simulink model "MDCC"  (R2021b)
settings: Solver=FixedStepDiscrete  StartTime=0.0  StopTime=10.0  FixedStep=0.0001  RelTol=1e-3
model workspace (MATLAB code in the model file):
  | cmdLim = Simulink.Parameter;
  | cmdLim.Value = 15;
  | cmdLim.Description = 'Limit for controlling the maximum surface command angle.';
  | cmdLim.Min = 0;
  | cmdLim.Max = 90;
  | cmdLim.DocUnits = 'deg';
  | 
  | dispGain = Simulink.Parameter;
  | dispGain.Value = 0.75;
  | dispGain.Description = 'Gain applied to the displacement error.';
  | dispGain.Min = 0;
  | dispGain.Max = [];
  | dispGain.DocUnits = 'deg/sec/deg';
  | 
  | dispLim = Simulink.Parameter;
  | dispLim.Value = 30;
  | dispLim.Description = 'Limit for controlling the maximum commanded angle.';
  | dispLim.Min = 0;
  | dispLim.Max = 180;
  | dispLim.DocUnits = 'deg';
  | 
  | intGain = Simulink.Parameter;
  | intGain.Value = 0.5;
  | intGain.Description = 'Gain applied to the integral error.';
  | intGain.Min = 0;
  | intGain.Max = [];
  | intGain.DocUnits = 'deg/sec/deg/sec';
  | 
  | intLim = Simulink.Parameter;
  | intLim.Value = 5;
  | intLim.Description = 'Limit for controlling the maximum commanded angle.';
  | intLim.Min = 0;
  | intLim.Max = 90;
  | intLim.DocUnits = 'deg';
  | 
  | rateGain = Simulink.Parameter;
  | rateGain.Value = 2;
  | rateGain.Description = 'Gain applied to the rate error.';
  | rateGain.Min = 0;
  | rateGain.Max = [];
  | rateGain.DocUnits = 'deg/deg/sec';
  | 
  | rateLim = Simulink.Parameter;
  | rateLim.Value = 6;
  | rateLim.Description = 'Limit for controlling the maximum commanded angle.';
  | rateLim.Min = 0;
  | rateLim.Max = 180;
  | rateLim.DocUnits = 'deg/sec';
  | 
  | hdgGain = Simulink.Parameter;
  | hdgGain.Value = 0.015;
values from neighbouring files (symbols this model uses):
  KfDeadCompen_SetDeltaTime_us = myPackage.Parameter    [DeadCompen.m]
  Ts = 5E-6    (= 5e-06)    [iPMSM_data.m]
  VbDeadComp_SwtUseIsttrDes_flg = myPackage.Parameter    [DeadCompen.m]
  VfDeadCompen_ISttrDdeThdSwt_A = myPackage.Parameter    [DeadCompen.m]
  VfDeadCompen_ISttrIgbtThdSwt_A = myPackage.Parameter    [DeadCompen.m]
  VfDeadCompen_rDdeISttrHi_R = myPackage.Parameter    [DeadCompen.m]
  VfDeadCompen_rDdeISttrLo_R = myPackage.Parameter    [DeadCompen.m]
  VfDeadCompen_rIgbtISttrHi_R = myPackage.Parameter    [DeadCompen.m]
  VfDeadCompen_rIgbtISttrLo_R = myPackage.Parameter    [DeadCompen.m]
  VfDeadCompen_uDdeISttrHi_V = myPackage.Parameter    [DeadCompen.m]
  VfDeadCompen_uDdeISttrLo_V = myPackage.Parameter    [DeadCompen.m]
  VfDeadCompen_uIgbtISttrHi_V = myPackage.Parameter    [DeadCompen.m]
  VfDeadCompen_uIgbtISttrLo_V = myPackage.Parameter    [DeadCompen.m]
undefined symbols (not defined in the file or in its folder): CosTable12bit_Y, GLBCal_GLBCal_Kf_DCLinkOverVolErrThd_V, GLBCal_GLBCal_Kf_DCLinkUnderVolErrThd_V, GLBCal_GLBCal_Kf_EquiLd_NULL, GLBCal_GLBCal_Kf_EquiLq_NULL, GLBCal_GLBCal_Kf_MotorRatedSpeed_rpm, GLBCal_GLBCal_Kf_MotorSpeedHysteresis_Coef, GLBCal_Ke_MotorPolePairsNum_NULL, IoHwAbOpArg_PwmDutyCyclePhU_NULL, IoHwAbOpArg_PwmDutyCyclePhV_NULL, IoHwAbOpArg_PwmDutyCyclePhW_NULL, IoHwAbOpArg_PwmOutputEn, KbMDCC_DeadTimeCompEn_flg, KbMDCC_MCF_flgHarmInIsdqTab11ZR_flg, KbMDCC_MCF_flgHarmInIsdqTab13ZR_flg, KbMDCC_MCF_flgHarmInIsdqTab5ZR_flg, KbMDCC_MCF_flgHarmInIsdqTab7ZR_flg, KbMDCC_MCF_flgHarmInject_flg, KbMDCC_SetEAngleEn_flg, KbMDCC_UdUqFwOmit_flg, KfDeadCompen_CpPeriodTimesT_NULL, KfMDCC_ActiveDischargeIdCurVal_A, KfMDCC_ActiveDischargeIqCurVal_A, KfMDCC_DCLinkVolRate_coef, KfMDCC_DebugEAngleInit_rad, KfMDCC_DebugUalphaVolCmd_V, KfMDCC_DebugUbetaVolCmd_V, KfMDCC_DebugUdCmd_V, KfMDCC_DebugUqCmd_V, KfMDCC_DebugUsCmd_V, KfMDCC_DebugUsRate_V, KfMDCC_IMCResp_NULL, KfMDCC_IMCStab_NULL, KfMDCC_InvParkCpPeriodTimesT_NULL, KfMDCC_MCF_CircAge_NULL, KfMDCC_MCF_flgUse11Harm_flg, KfMDCC_MCF_flgUse13Harm_flg, KfMDCC_MCF_flgUse5Harm_flg, KfMDCC_MCF_flgUse7Harm_flg, KfMDCC_MCF_Harm1113FLParamSpeedThrd_rads, KfMDCC_MCF_Harm57FLParamSpeedThrd_rads, KfMDCC_MCF_HarmcofFltN_NULL, KfMDCC_MCF_HarmCpnAg_NULL, KfMDCC_MCF_HarmfLParaHigh_coef, KfMDCC_MCF_HarmfLParaLow_coef, KfMDCC_MCF_HarmIn1113ZRY_Trq_Nm, KfMDCC_MCF_HarmIn11_SpdLimHigh_rads, KfMDCC_MCF_HarmIn11_SpdLimLow_rads, KfMDCC_MCF_HarmIn11ZRY_Isd_A, KfMDCC_MCF_HarmIn11ZRY_Isq_A, KfMDCC_MCF_HarmIn13_SpdLimHigh_rads, KfMDCC_MCF_HarmIn13_SpdLimLow_rads, KfMDCC_MCF_HarmIn13ZRY_Isd_A, KfMDCC_MCF_HarmIn13ZRY_Isq_A, KfMDCC_MCF_HarmIn57ZRY_Trq_Nm, KfMDCC_MCF_HarmIn5_SpdLimHigh_rads, KfMDCC_MCF_HarmIn5_SpdLimLow_rads, KfMDCC_MCF_HarmIn5ZRY_Isd_A, KfMDCC_MCF_HarmIn5ZRY_Isq_A, KfMDCC_MCF_HarmIn7_SpdLimHigh_rads ... (+47)
libraries: simulink x40, PMSM_Library x3, mcbcontrolslib x1
(part 7 of 8)

== system MDCC/DoCurCtr_sys/MDCC/UdUqCalc_Sys/MDCC_MCF_Sys/Enabled Subsystem/Subsystem1/Park5/Subsystem ==
  In1 : Inport
  MCF_dtPWM : Inport  Port=2
  dB_Harm : Inport  Port=3
  Add : Sum
  Add1 : Sum  Inputs=-+
  Add2 : Sum
  Constant1 : Constant  OutDataTypeStr=single
  Constant2 : Constant  Value=2*pi  OutDataTypeStr=single
  Constant4 : Constant  OutDataTypeStr=single
  Divide{,1..3} (4 alike) : Product  Inputs=**
  Divide4 : Product  Inputs=*/
  Unit Delay : UnitDelay  SampleTime=-1  HasFrameUpgradeWarning=on
  Out1 : Outport
  wires:
  Add/1 -> Out1/1, Unit Delay/1
  Divide/1 -> Add/1
  Constant1/1 -> Add1/2
  Add1/1 -> Divide1/1
  Constant2/1 -> Divide2/1
  MCF_dtPWM/1 -> Divide2/2
  dB_Harm/1 -> Divide3/1
  Divide2/1 -> Divide3/2
  Divide3/1 -> Add2/2
  Constant4/1 -> Add2/1, Divide4/1
  Add2/1 -> Divide4/2
  Divide4/1 -> Divide/2, Add1/1
  In1/1 -> Divide1/2
  Divide1/1 -> Add/2
  Unit Delay/1 -> Divide/1

== system MDCC/DoCurCtr_sys/MDCC/UdUqCalc_Sys/MDCC_MCF_Sys/Enabled Subsystem/Subsystem1/Park5/Subsystem1 ==
  dB_Harm : Inport
  MCF_dtPWM : Inport  Port=2
  In1 : Inport  Port=3
  Add : Sum
  Add1 : Sum  Inputs=-+
  Add2 : Sum
  Constant1 : Constant  OutDataTypeStr=single
  Constant2 : Constant  Value=2*pi  OutDataTypeStr=single
  Constant4 : Constant  OutDataTypeStr=single
  Divide{,1..3} (4 alike) : Product  Inputs=**
  Divide4 : Product  Inputs=*/
  Unit Delay : UnitDelay  SampleTime=-1  HasFrameUpgradeWarning=on
  Out1 : Outport
  wires:
  Unit Delay/1 -> Divide/1
  Divide1/1 -> Add/2
  In1/1 -> Divide1/2
  Divide4/1 -> Add1/1, Divide/2
  Add2/1 -> Divide4/2
  Constant4/1 -> Divide4/1, Add2/1
  Divide3/1 -> Add2/2
  Divide2/1 -> Divide3/2
  dB_Harm/1 -> Divide3/1
  MCF_dtPWM/1 -> Divide2/2
  Constant2/1 -> Divide2/1
  Add1/1 -> Divide1/1
  Constant1/1 -> Add1/2
  Divide/1 -> Add/1
  Add/1 -> Unit Delay/1, Out1/1

== system MDCC/DoCurCtr_sys/MDCC/UdUqCalc_Sys/MDCC_MCF_Sys/Enabled Subsystem/Subsystem1/Park7/Subsystem ==
  In1 : Inport
  MCF_dtPWM : Inport  Port=2
  dB_Harm : Inport  Port=3
  Add : Sum
  Add1 : Sum  Inputs=-+
  Add2 : Sum
  Constant1 : Constant  OutDataTypeStr=single
  Constant2 : Constant  Value=2*pi  OutDataTypeStr=single
  Constant4 : Constant  OutDataTypeStr=single
  Divide{,1..3} (4 alike) : Product  Inputs=**
  Divide4 : Product  Inputs=*/
  Unit Delay : UnitDelay  SampleTime=-1  HasFrameUpgradeWarning=on
  Out1 : Outport
  wires:
  Add/1 -> Out1/1, Unit Delay/1
  Divide/1 -> Add/1
  Constant1/1 -> Add1/2
  Add1/1 -> Divide1/1
  Constant2/1 -> Divide2/1
  MCF_dtPWM/1 -> Divide2/2
  dB_Harm/1 -> Divide3/1
  Divide2/1 -> Divide3/2
  Divide3/1 -> Add2/2
  Constant4/1 -> Add2/1, Divide4/1
  Add2/1 -> Divide4/2
  Divide4/1 -> Divide/2, Add1/1
  In1/1 -> Divide1/2
  Divide1/1 -> Add/2
  Unit Delay/1 -> Divide/1

== system MDCC/DoCurCtr_sys/MDCC/UdUqCalc_Sys/MDCC_MCF_Sys/Enabled Subsystem/Subsystem1/Park7/Subsystem1 ==
  dB_Harm : Inport
  MCF_dtPWM : Inport  Port=2
  In1 : Inport  Port=3
  Add : Sum
  Add1 : Sum  Inputs=-+
  Add2 : Sum
  Constant1 : Constant  OutDataTypeStr=single
  Constant2 : Constant  Value=2*pi  OutDataTypeStr=single
  Constant4 : Constant  OutDataTypeStr=single
  Divide{,1..3} (4 alike) : Product  Inputs=**
  Divide4 : Product  Inputs=*/
  Unit Delay : UnitDelay  SampleTime=-1  HasFrameUpgradeWarning=on
  Out1 : Outport
  wires:
  Unit Delay/1 -> Divide/1
  Divide1/1 -> Add/2
  In1/1 -> Divide1/2
  Divide4/1 -> Add1/1, Divide/2
  Add2/1 -> Divide4/2
  Constant4/1 -> Divide4/1, Add2/1
  Divide3/1 -> Add2/2
  Divide2/1 -> Divide3/2
  dB_Harm/1 -> Divide3/1
  MCF_dtPWM/1 -> Divide2/2
  Constant2/1 -> Divide2/1
  Add1/1 -> Divide1/1
  Constant1/1 -> Add1/2
  Divide/1 -> Add/1
  Add/1 -> Unit Delay/1, Out1/1

== system MDCC/DoCurCtr_sys/MDCC/UdUqCalc_Sys/MDCC_MCF_Sys/Enabled Subsystem/Subsystem1/Subsystem/LookUpEAngleCosSin1 ==
  VuMDCC_MotorPositionCnt_NULL : Inport  OutMin=[0]  OutMax=[4095]
  Constant2 : Constant  Value=CosTable12bit_Y
  Constant3 : Constant  Value=SinTable12bit_Y
  Direct Lookup Table (n-D) : LookupNDDirect  NumberOfTableDimensions=1  TableIsInput=on  Table=[4 5 6]  TableMax=[4096]
  Direct Lookup Table (n-D)1 : LookupNDDirect  NumberOfTableDimensions=1  TableIsInput=on  Table=[4 5 6]  TableMax=[4096]
  VfMDCC_EAngleCos_NULL : Outport
  VfMDCC_EAngleSin_NULL : Outport  Port=2
  wires:
  VuMDCC_MotorPositionCnt_NULL/1 -> Direct Lookup Table (n-D)/1, Direct Lookup Table (n-D)1/1
  Direct Lookup Table (n-D)/1 -> VfMDCC_EAngleCos_NULL/1
  Direct Lookup Table (n-D)1/1 -> VfMDCC_EAngleSin_NULL/1
  Constant2/1 -> Direct Lookup Table (n-D)/2
  Constant3/1 -> Direct Lookup Table (n-D)1/2

== system MDCC/DoCurCtr_sys/MDCC/UdUqCalc_Sys/MDCC_MCF_Sys/Enabled Subsystem/Subsystem1/Subsystem/LookUpEAngleCosSin2 ==
  VuMDCC_MotorPositionCnt_NULL : Inport  OutMin=[0]  OutMax=[4095]
  Constant2 : Constant  Value=CosTable12bit_Y
  Constant3 : Constant  Value=SinTable12bit_Y
  Direct Lookup Table (n-D) : LookupNDDirect  NumberOfTableDimensions=1  TableIsInput=on  Table=[4 5 6]  TableMax=[4096]
  Direct Lookup Table (n-D)1 : LookupNDDirect  NumberOfTableDimensions=1  TableIsInput=on  Table=[4 5 6]  TableMax=[4096]
  VfMDCC_EAngleCos_NULL : Outport
  VfMDCC_EAngleSin_NULL : Outport  Port=2
  wires:
  VuMDCC_MotorPositionCnt_NULL/1 -> Direct Lookup Table (n-D)/1, Direct Lookup Table (n-D)1/1
  Direct Lookup Table (n-D)/1 -> VfMDCC_EAngleCos_NULL/1
  Direct Lookup Table (n-D)1/1 -> VfMDCC_EAngleSin_NULL/1
  Constant2/1 -> Direct Lookup Table (n-D)/2
  Constant3/1 -> Direct Lookup Table (n-D)1/2

== system MDCC/DoCurCtr_sys/MDCC/UdUqCalc_Sys/MDCC_MCF_Sys/Enabled Subsystem/Subsystem1/Subsystem/LookUpEAngleCosSin3 ==
  VuMDCC_MotorPositionCnt_NULL : Inport  OutMin=[0]  OutMax=[4095]
  Constant2 : Constant  Value=CosTable12bit_Y
  Constant3 : Constant  Value=SinTable12bit_Y
  Direct Lookup Table (n-D) : LookupNDDirect  NumberOfTableDimensions=1  TableIsInput=on  Table=[4 5 6]  TableMax=[4096]
  Direct Lookup Table (n-D)1 : LookupNDDirect  NumberOfTableDimensions=1  TableIsInput=on  Table=[4 5 6]  TableMax=[4096]
  VfMDCC_EAngleCos_NULL : Outport
  VfMDCC_EAngleSin_NULL : Outport  Port=2
  wires:
  VuMDCC_MotorPositionCnt_NULL/1 -> Direct Lookup Table (n-D)/1, Direct Lookup Table (n-D)1/1
  Direct Lookup Table (n-D)/1 -> VfMDCC_EAngleCos_NULL/1
  Direct Lookup Table (n-D)1/1 -> VfMDCC_EAngleSin_NULL/1
  Constant2/1 -> Direct Lookup Table (n-D)/2
  Constant3/1 -> Direct Lookup Table (n-D)1/2

== system MDCC/DoCurCtr_sys/MDCC/UdUqCalc_Sys/MDCC_MCF_Sys/Enabled Subsystem/Subsystem1/Subsystem/LookUpEAngleCosSin5 ==
  VuMDCC_MotorPositionCnt_NULL : Inport  OutMin=[0]  OutMax=[4095]
  Constant2 : Constant  Value=CosTable12bit_Y
  Constant3 : Constant  Value=SinTable12bit_Y
  Direct Lookup Table (n-D) : LookupNDDirect  NumberOfTableDimensions=1  TableIsInput=on  Table=[4 5 6]  TableMax=[4096]
  Direct Lookup Table (n-D)1 : LookupNDDirect  NumberOfTableDimensions=1  TableIsInput=on  Table=[4 5 6]  TableMax=[4096]
  VfMDCC_EAngleCos_NULL : Outport
  VfMDCC_EAngleSin_NULL : Outport  Port=2
  wires:
  VuMDCC_MotorPositionCnt_NULL/1 -> Direct Lookup Table (n-D)/1, Direct Lookup Table (n-D)1/1
  Direct Lookup Table (n-D)/1 -> VfMDCC_EAngleCos_NULL/1
  Direct Lookup Table (n-D)1/1 -> VfMDCC_EAngleSin_NULL/1
  Constant2/1 -> Direct Lookup Table (n-D)/2
  Constant3/1 -> Direct Lookup Table (n-D)1/2

== system MDCC/DoCurCtr_sys/MDCC/UdUqCalc_Sys/MDCC_MCF_Sys/Enabled Subsystem/Subsystem2/Mcf_AgTranCalc11/LookUpEAngleCosSin2 ==
  VuMDCC_MotorPositionCnt_NULL : Inport  OutMin=[0]  OutMax=[4095]
  Constant2 : Constant  Value=CosTable12bit_Y
  Constant3 : Constant  Value=SinTable12bit_Y
  Direct Lookup Table (n-D) : LookupNDDirect  NumberOfTableDimensions=1  TableIsInput=on  Table=[4 5 6]  TableMax=[4096]
  Direct Lookup Table (n-D)1 : LookupNDDirect  NumberOfTableDimensions=1  TableIsInput=on  Table=[4 5 6]  TableMax=[4096]
  VfMDCC_EAngleCos_NULL : Outport
  VfMDCC_EAngleSin_NULL : Outport  Port=2
  wires:
  VuMDCC_MotorPositionCnt_NULL/1 -> Direct Lookup Table (n-D)/1, Direct Lookup Table (n-D)1/1
  Direct Lookup Table (n-D)/1 -> VfMDCC_EAngleCos_NULL/1
  Direct Lookup Table (n-D)1/1 -> VfMDCC_EAngleSin_NULL/1
  Constant2/1 -> Direct Lookup Table (n-D)/2
  Constant3/1 -> Direct Lookup Table (n-D)1/2

== system MDCC/DoCurCtr_sys/MDCC/UdUqCalc_Sys/MDCC_MCF_Sys/Enabled Subsystem/Subsystem2/Mcf_AgTranCalc13/LookUpEAngleCosSin2 ==
  VuMDCC_MotorPositionCnt_NULL : Inport  OutMin=[0]  OutMax=[4095]
  Constant2 : Constant  Value=CosTable12bit_Y
  Constant3 : Constant  Value=SinTable12bit_Y
  Direct Lookup Table (n-D) : LookupNDDirect  NumberOfTableDimensions=1  TableIsInput=on  Table=[4 5 6]  TableMax=[4096]
  Direct Lookup Table (n-D)1 : LookupNDDirect  NumberOfTableDimensions=1  TableIsInput=on  Table=[4 5 6]  TableMax=[4096]
  VfMDCC_EAngleCos_NULL : Outport
  VfMDCC_EAngleSin_NULL : Outport  Port=2
  wires:
  VuMDCC_MotorPositionCnt_NULL/1 -> Direct Lookup Table (n-D)/1, Direct Lookup Table (n-D)1/1
  Direct Lookup Table (n-D)/1 -> VfMDCC_EAngleCos_NULL/1
  Direct Lookup Table (n-D)1/1 -> VfMDCC_EAngleSin_NULL/1
  Constant2/1 -> Direct Lookup Table (n-D)/2
  Constant3/1 -> Direct Lookup Table (n-D)1/2

== system MDCC/DoCurCtr_sys/MDCC/UdUqCalc_Sys/MDCC_MCF_Sys/Enabled Subsystem/Subsystem2/Mcf_AgTranCalc5/LookUpEAngleCosSin2 ==
  VuMDCC_MotorPositionCnt_NULL : Inport  OutMin=[0]  OutMax=[4095]
  Constant2 : Constant  Value=CosTable12bit_Y
  Constant3 : Constant  Value=SinTable12bit_Y
  Direct Lookup Table (n-D) : LookupNDDirect  NumberOfTableDimensions=1  TableIsInput=on  Table=[4 5 6]  TableMax=[4096]
  Direct Lookup Table (n-D)1 : LookupNDDirect  NumberOfTableDimensions=1  TableIsInput=on  Table=[4 5 6]  TableMax=[4096]
  VfMDCC_EAngleCos_NULL : Outport
  VfMDCC_EAngleSin_NULL : Outport  Port=2
  wires:
  VuMDCC_MotorPositionCnt_NULL/1 -> Direct Lookup Table (n-D)/1, Direct Lookup Table (n-D)1/1
  Direct Lookup Table (n-D)/1 -> VfMDCC_EAngleCos_NULL/1
  Direct Lookup Table (n-D)1/1 -> VfMDCC_EAngleSin_NULL/1
  Constant2/1 -> Direct Lookup Table (n-D)/2
  Constant3/1 -> Direct Lookup Table (n-D)1/2

== system MDCC/DoCurCtr_sys/MDCC/UdUqCalc_Sys/MDCC_MCF_Sys/Enabled Subsystem/Subsystem2/Mcf_AgTranCalc7/LookUpEAngleCosSin2 ==
  VuMDCC_MotorPositionCnt_NULL : Inport  OutMin=[0]  OutMax=[4095]
  Constant2 : Constant  Value=CosTable12bit_Y
  Constant3 : Constant  Value=SinTable12bit_Y
  Direct Lookup Table (n-D) : LookupNDDirect  NumberOfTableDimensions=1  TableIsInput=on  Table=[4 5 6]  TableMax=[4096]
  Direct Lookup Table (n-D)1 : LookupNDDirect  NumberOfTableDimensions=1  TableIsInput=on  Table=[4 5 6]  TableMax=[4096]
  VfMDCC_EAngleCos_NULL : Outport
  VfMDCC_EAngleSin_NULL : Outport  Port=2
  wires:
  VuMDCC_MotorPositionCnt_NULL/1 -> Direct Lookup Table (n-D)/1, Direct Lookup Table (n-D)1/1
  Direct Lookup Table (n-D)/1 -> VfMDCC_EAngleCos_NULL/1
  Direct Lookup Table (n-D)1/1 -> VfMDCC_EAngleSin_NULL/1
  Constant2/1 -> Direct Lookup Table (n-D)/2
  Constant3/1 -> Direct Lookup Table (n-D)1/2

== system MDCC/DoCurCtr_sys/MDCC/UdUqCalc_Sys/MDCC_MCF_Sys/Enabled Subsystem/Subsystem2/Subsystem/First_LowPass ==
  MCF_n : Inport
  Add : Sum  Inputs=-+
  Add1 : Sum
  CAL_MCF_HarmcofFltN_f32 : Constant  Value=KfMDCC_MCF_HarmcofFltN_NULL
  Constant : Constant  OutDataTypeStr=single
  Product : Product
  Product1 : Product
  Unit Delay : UnitDelay  SampleTime=-1  HasFrameUpgradeWarning=on
  MCF_nFlt : Outport
  wires:
  MCF_n/1 -> Product/1
  CAL_MCF_HarmcofFltN_f32/1 -> Product/2, Add/1
  Constant/1 -> Add/2
  Add/1 -> Product1/1
  Product1/1 -> Add1/2
  Product/1 -> Add1/1
  Add1/1 -> Unit Delay/1, MCF_nFlt/1
  Unit Delay/1 -> Product1/2

== system MDCC/DoCurCtr_sys/MDCC/SVM_Calc/DeadComp_Sys/DeadTime_Calc/Tavon_Calc/ia/uDdeCalc/If Action Subsystem ==
  iPhaseAbs : Inport
  Action Port : ActionPort  ActionPortLabel=if(u1 == 1)
  Add : Sum
  Constant : Constant  Value=VfDeadCompen_uDdeISttrLo_V
  Constant1 : Constant  Value=VfDeadCompen_rDdeISttrLo_R
  Product : Product
  UDde : Outport
  wires:
  Constant/1 -> Add/1
  Constant1/1 -> Product/1
  iPhaseAbs/1 -> Product/2
  Product/1 -> Add/2
  Add/1 -> UDde/1

== system MDCC/DoCurCtr_sys/MDCC/SVM_Calc/DeadComp_Sys/DeadTime_Calc/Tavon_Calc/ia/uDdeCalc/If Action Subsystem1 ==
  iPhaseAbs : Inport
  Action Port : ActionPort  ActionPortLabel=else
  Add : Sum
  Constant : Constant  Value=VfDeadCompen_uDdeISttrHi_V
  Constant1 : Constant  Value=VfDeadCompen_rDdeISttrHi_R
  Product : Product
  UDde : Outport
  wires:
  iPhaseAbs/1 -> Product/2
  Constant/1 -> Add/1
  Add/1 -> UDde/1
  Constant1/1 -> Product/1
  Product/1 -> Add/2

== system MDCC/DoCurCtr_sys/MDCC/SVM_Calc/DeadComp_Sys/DeadTime_Calc/Tavon_Calc/ia/uIgbtCalc/If Action Subsystem ==
  iPhaseAbs : Inport
  Action Port : ActionPort  ActionPortLabel=if(u1 == 0)
  Add : Sum
  Constant : Constant  Value=VfDeadCompen_uIgbtISttrLo_V
  Constant1 : Constant  Value=VfDeadCompen_rIgbtISttrLo_R
  Product : Product
  uIgbt : Outport
  wires:
  Constant/1 -> Add/1
  Constant1/1 -> Product/1
  iPhaseAbs/1 -> Product/2
  Product/1 -> Add/2
  Add/1 -> uIgbt/1

== system MDCC/DoCurCtr_sys/MDCC/SVM_Calc/DeadComp_Sys/DeadTime_Calc/Tavon_Calc/ia/uIgbtCalc/If Action Subsystem1 ==
  iPhaseAbs : Inport
  Action Port : ActionPort  ActionPortLabel=else
  Add : Sum
  Constant : Constant  Value=VfDeadCompen_uIgbtISttrHi_V
  Constant1 : Constant  Value=VfDeadCompen_rIgbtISttrHi_R
  Product : Product
  uIgbt : Outport
  wires:
  iPhaseAbs/1 -> Product/2
  Constant/1 -> Add/1
  Add/1 -> uIgbt/1
  Constant1/1 -> Product/1
  Product/1 -> Add/2

== system MDCC/DoCurCtr_sys/MDCC/SVM_Calc/DeadComp_Sys/DeadTime_Calc/Tavon_Calc/ib/uDdeCalc/If Action Subsystem ==
  iPhaseAbs : Inport
  Action Port : ActionPort  ActionPortLabel=if(u1 == 1)
  Add : Sum
  Constant : Constant  Value=VfDeadCompen_uDdeISttrLo_V
  Constant1 : Constant  Value=VfDeadCompen_rDdeISttrLo_R
  Product : Product
  UDde : Outport
  wires:
  Constant/1 -> Add/1
  Constant1/1 -> Product/1
  iPhaseAbs/1 -> Product/2
  Product/1 -> Add/2
  Add/1 -> UDde/1

== system MDCC/DoCurCtr_sys/MDCC/SVM_Calc/DeadComp_Sys/DeadTime_Calc/Tavon_Calc/ib/uDdeCalc/If Action Subsystem1 ==
  iPhaseAbs : Inport
  Action Port : ActionPort  ActionPortLabel=else
  Add : Sum
  Constant : Constant  Value=VfDeadCompen_uDdeISttrHi_V
  Constant1 : Constant  Value=VfDeadCompen_rDdeISttrHi_R
  Product : Product
  UDde : Outport
  wires:
  iPhaseAbs/1 -> Product/2
  Constant/1 -> Add/1
  Add/1 -> UDde/1
  Constant1/1 -> Product/1
  Product/1 -> Add/2

== system MDCC/DoCurCtr_sys/MDCC/SVM_Calc/DeadComp_Sys/DeadTime_Calc/Tavon_Calc/ib/uIgbtCalc/If Action Subsystem ==
  iPhaseAbs : Inport
  Action Port : ActionPort  ActionPortLabel=if(u1 == 0)
  Add : Sum
  Constant : Constant  Value=VfDeadCompen_uIgbtISttrLo_V
  Constant1 : Constant  Value=VfDeadCompen_rIgbtISttrLo_R
  Product : Product
  uIgbt : Outport
  wires:
  Constant/1 -> Add/1
  Constant1/1 -> Product/1
  iPhaseAbs/1 -> Product/2
  Product/1 -> Add/2
  Add/1 -> uIgbt/1

== system MDCC/DoCurCtr_sys/MDCC/SVM_Calc/DeadComp_Sys/DeadTime_Calc/Tavon_Calc/ib/uIgbtCalc/If Action Subsystem1 ==
  iPhaseAbs : Inport
  Action Port : ActionPort  ActionPortLabel=else
  Add : Sum
  Constant : Constant  Value=VfDeadCompen_uIgbtISttrHi_V
  Constant1 : Constant  Value=VfDeadCompen_rIgbtISttrHi_R
  Product : Product
  uIgbt : Outport
  wires:
  iPhaseAbs/1 -> Product/2
  Constant/1 -> Add/1
  Add/1 -> uIgbt/1
  Constant1/1 -> Product/1
  Product/1 -> Add/2

== system MDCC/DoCurCtr_sys/MDCC/SVM_Calc/DeadComp_Sys/DeadTime_Calc/Tavon_Calc/ic/uDdeCalc/If Action Subsystem ==
  iPhaseAbs : Inport
  Action Port : ActionPort  ActionPortLabel=if(u1 == 1)
  Add : Sum
  Constant : Constant  Value=VfDeadCompen_uDdeISttrLo_V
  Constant1 : Constant  Value=VfDeadCompen_rDdeISttrLo_R
  Product : Product
  UDde : Outport
  wires:
  Constant/1 -> Add/1
  Constant1/1 -> Product/1
  iPhaseAbs/1 -> Product/2
  Product/1 -> Add/2
  Add/1 -> UDde/1

== system MDCC/DoCurCtr_sys/MDCC/SVM_Calc/DeadComp_Sys/DeadTime_Calc/Tavon_Calc/ic/uDdeCalc/If Action Subsystem1 ==
  iPhaseAbs : Inport
  Action Port : ActionPort  ActionPortLabel=else
  Add : Sum
  Constant : Constant  Value=VfDeadCompen_uDdeISttrHi_V
  Constant1 : Constant  Value=VfDeadCompen_rDdeISttrHi_R
  Product : Product
  UDde : Outport
  wires:
  iPhaseAbs/1 -> Product/2
  Constant/1 -> Add/1
  Add/1 -> UDde/1
  Constant1/1 -> Product/1
  Product/1 -> Add/2

== system MDCC/DoCurCtr_sys/MDCC/SVM_Calc/DeadComp_Sys/DeadTime_Calc/Tavon_Calc/ic/uIgbtCalc/If Action Subsystem ==
  iPhaseAbs : Inport
  Action Port : ActionPort  ActionPortLabel=if(u1 == 0)
  Add : Sum
  Constant : Constant  Value=VfDeadCompen_uIgbtISttrLo_V
  Constant1 : Constant  Value=VfDeadCompen_rIgbtISttrLo_R
  Product : Product
  uIgbt : Outport
  wires:
  Constant/1 -> Add/1
  Constant1/1 -> Product/1
  iPhaseAbs/1 -> Product/2
  Product/1 -> Add/2
  Add/1 -> uIgbt/1

== system MDCC/DoCurCtr_sys/MDCC/SVM_Calc/DeadComp_Sys/DeadTime_Calc/Tavon_Calc/ic/uIgbtCalc/If Action Subsystem1 ==
  iPhaseAbs : Inport
  Action Port : ActionPort  ActionPortLabel=else
  Add : Sum
  Constant : Constant  Value=VfDeadCompen_uIgbtISttrHi_V
  Constant1 : Constant  Value=VfDeadCompen_rIgbtISttrHi_R
  Product : Product
  uIgbt : Outport
  wires:
  iPhaseAbs/1 -> Product/2
  Constant/1 -> Add/1
  Add/1 -> uIgbt/1
  Constant1/1 -> Product/1
  Product/1 -> Add/2

== system MDCC/DoCurCtr_sys/MDCC/SVM_Calc/MDSA/SVM_PU/T1_T2_Calc/Subsystem2/If Action Subsystem2/If Action Subsystem2 ==
  T4_m : Inport
  T6_m : Inport  Port=2
  delta : Inport  Port=3
  Action Port : ActionPort  ActionPortLabel=if(u1 ~= 0)
  Add : Sum
  Add1 : Sum  Inputs=-+
  Constant : Constant  OutDataTypeStr=single
  Constant1 : Constant  Value=0  OutDataTypeStr=single
  Demux : Demux  Outputs=2
  Mux : Mux  Inputs=2
  Mux1 : Mux  Inputs=2
  Relational Operator : RelationalOperator  Operator=<=  OutDataTypeStr=boolean  RndMeth=Simplest
  Switch : Switch  Criteria=u2 > Threshold
  T1 : Outport
  T2 : Outport  Port=2
  wires:
  T6_m/1 -> Add1/2, Relational Operator/1
  delta/1 -> Add/1, Add1/1, Relational Operator/2
  Relational Operator/1 -> Switch/2
  Constant/1 -> Mux/1
  Constant1/1 -> Mux/2
  Mux/1 -> Switch/1
  T4_m/1 -> Add/2
  Add/1 -> Mux1/1
  Add1/1 -> Mux1/2
  Mux1/1 -> Switch/3
  Switch/1 -> Demux/1
  Demux/1 -> T1/1
  Demux/2 -> T2/1

== system MDCC/DoCurCtr_sys/MDCC/SVM_Calc/MDSA/SVM_PU/T1_T2_Calc/Subsystem2/If Action Subsystem2/If Action Subsystem3 ==
  T4_m : Inport
  T6_m : Inport  Port=2
  delta : Inport  Port=3
  Action Port : ActionPort  ActionPortLabel=else
  Add : Sum
  Add1 : Sum  Inputs=-+
  Constant : Constant  OutDataTypeStr=single
  Constant1 : Constant  Value=0  OutDataTypeStr=single
  Demux : Demux  Outputs=2
  Mux : Mux  Inputs=2
  Mux1 : Mux  Inputs=2
  Relational Operator : RelationalOperator  Operator=<=  OutDataTypeStr=boolean  RndMeth=Simplest
  Switch : Switch  Criteria=u2 > Threshold
  T1 : Outport
  T2 : Outport  Port=2
  wires:
  Mux1/1 -> Switch/3
  delta/1 -> Add/1, Add1/1, Relational Operator/2
  Add1/1 -> Mux1/2
  Mux/1 -> Switch/1
  Relational Operator/1 -> Switch/2
  Switch/1 -> Demux/1
  Constant1/1 -> Mux/2
  Add/1 -> Mux1/1
  Constant/1 -> Mux/1
  T4_m/1 -> Add1/2, Relational Operator/1
  T6_m/1 -> Add/2
  Demux/2 -> T1/1
  Demux/1 -> T2/1

== system MDCC/DoCurCtr_sys/MDCC/SVM_Calc/MDSA/SVPWM/vIntp_PWMFOC_CalTriCompValue/CalTabc/Cal_T1T2/Sec1 ==
  Bus_XYZ_IN : Inport
  Action Port : ActionPort  ActionPortLabel=case [ 1 ]:
  Bus Creator1 : BusCreator  Inputs=2
  Bus Selector : BusSelector  OutputSignals=Z,Y
  Signal Conversion : SignalConversion  OverrideOpt=off
  Signal Conversion1 : SignalConversion  OverrideOpt=off
  Bus_T1T2 : Outport
  wires:
  Signal Conversion1/1 -> Bus Creator1/2
  Signal Conversion/1 -> Bus Creator1/1
  Bus Selector/2 -> Signal Conversion1/1  "<Y>"
  Bus Selector/1 -> Signal Conversion/1  "<Z>"
  Bus_XYZ_IN/1 -> Bus Selector/1
  Bus Creator1/1 -> Bus_T1T2/1

== system MDCC/DoCurCtr_sys/MDCC/SVM_Calc/MDSA/SVPWM/vIntp_PWMFOC_CalTriCompValue/CalTabc/Cal_T1T2/Sec2 ==
  Bus_XYZ_IN : Inport
  Action Port : ActionPort  ActionPortLabel=case [ 2 ]:
  -1 : Constant  Value=-1
  Bus Creator1 : BusCreator  Inputs=2
  Bus Selector : BusSelector  OutputSignals=Y,X
  Data Type Conversion1 : DataTypeConversion
  Product1 : Product
  Signal Conversion1 : SignalConversion  OverrideOpt=off
  Bus_T1T2 : Outport
  wires:
  Signal Conversion1/1 -> Bus Creator1/1
  Bus_XYZ_IN/1 -> Bus Selector/1
  Bus Selector/1 -> Signal Conversion1/1  "<Y>"
  Bus Selector/2 -> Product1/1  "<X>"
  Bus Creator1/1 -> Bus_T1T2/1
  Product1/1 -> Bus Creator1/2
  Data Type Conversion1/1 -> Product1/2
  -1/1 -> Data Type Conversion1/1

== system MDCC/DoCurCtr_sys/MDCC/SVM_Calc/MDSA/SVPWM/vIntp_PWMFOC_CalTriCompValue/CalTabc/Cal_T1T2/Sec3 ==
  Bus_XYZ_IN : Inport
  Action Port : ActionPort  ActionPortLabel=case [ 3 ]:
  -1 : Constant  Value=-1
  Bus Creator1 : BusCreator  Inputs=2
  Bus Selector : BusSelector  OutputSignals=Z,X
  Data Type Conversion1 : DataTypeConversion
  Product1 : Product
  Signal Conversion1 : SignalConversion  OverrideOpt=off
  Bus_T1T2 : Outport
  wires:
  Signal Conversion1/1 -> Bus Creator1/2
  Data Type Conversion1/1 -> Product1/1
  Bus_XYZ_IN/1 -> Bus Selector/1
  Bus Creator1/1 -> Bus_T1T2/1
  Product1/1 -> Bus Creator1/1
  Bus Selector/1 -> Product1/2  "<Z>"
  -1/1 -> Data Type Conversion1/1
  Bus Selector/2 -> Signal Conversion1/1  "<X>"

== system MDCC/DoCurCtr_sys/MDCC/SVM_Calc/MDSA/SVPWM/vIntp_PWMFOC_CalTriCompValue/CalTabc/Cal_T1T2/Sec4 ==
  Bus_XYZ_IN : Inport
  Action Port : ActionPort  ActionPortLabel=case [ 4 ]:
  -1 : Constant  Value=-1
  Bus Creator1 : BusCreator  Inputs=2
  Bus Selector : BusSelector  OutputSignals=X,Z
  Data Type Conversion2 : DataTypeConversion
  Product1 : Product
  Signal Conversion1 : SignalConversion  OverrideOpt=off
  Bus_T1T2 : Outport
  wires:
  Signal Conversion1/1 -> Bus Creator1/2
  Data Type Conversion2/1 -> Product1/1
  Bus_XYZ_IN/1 -> Bus Selector/1
  Bus Selector/2 -> Signal Conversion1/1  "<Z>"
  Bus Creator1/1 -> Bus_T1T2/1
  Product1/1 -> Bus Creator1/1
  Bus Selector/1 -> Product1/2  "<X>"
  -1/1 -> Data Type Conversion2/1

== system MDCC/DoCurCtr_sys/MDCC/SVM_Calc/MDSA/SVPWM/vIntp_PWMFOC_CalTriCompValue/CalTabc/Cal_T1T2/Sec5 ==
  Bus_XYZ_IN : Inport
  Action Port : ActionPort  ActionPortLabel=case [ 5 ]:
  -1 : Constant  Value=-1
  Bus Creator1 : BusCreator  Inputs=2
  Bus Selector : BusSelector  OutputSignals=X,Y
  Data Type Conversion1 : DataTypeConversion
  Product1 : Product
  Signal Conversion1 : SignalConversion  OverrideOpt=off
  Bus_T1T2 : Outport
  wires:
  Signal Conversion1/1 -> Bus Creator1/1
  Bus_XYZ_IN/1 -> Bus Selector/1
  Bus Creator1/1 -> Bus_T1T2/1
  Product1/1 -> Bus Creator1/2
  Data Type Conversion1/1 -> Product1/2
  -1/1 -> Data Type Conversion1/1
  Bus Selector/2 -> Product1/1  "<Y>"
  Bus Selector/1 -> Signal Conversion1/1  "<X>"

== system MDCC/DoCurCtr_sys/MDCC/SVM_Calc/MDSA/SVPWM/vIntp_PWMFOC_CalTriCompValue/CalTabc/Cal_T1T2/Sec6 ==
  Bus_XYZ_IN : Inport
  Action Port : ActionPort  ActionPortLabel=case [ 6 ]:
  -1 : Constant  Value=-1
  -1_1 : Constant  Value=-1
  Bus Creator1 : BusCreator  Inputs=2
  Bus Selector : BusSelector  OutputSignals=Y,Z
  Data Type Conversion2 : DataTypeConversion
  Data Type Conversion3 : DataTypeConversion
  Product2 : Product
  Product3 : Product
  Bus_T1T2 : Outport
  wires:
  Data Type Conversion3/1 -> Product3/1
  Bus_XYZ_IN/1 -> Bus Selector/1
  Bus Creator1/1 -> Bus_T1T2/1
  Product3/1 -> Bus Creator1/1
  Product2/1 -> Bus Creator1/2
  Data Type Conversion2/1 -> Product2/2
  -1_1/1 -> Data Type Conversion2/1
  -1/1 -> Data Type Conversion3/1
  Bus Selector/1 -> Product3/2  "<Y>"
  Bus Selector/2 -> Product2/1  "<Z>"

== system MDCC/DoCurCtr_sys/MDCC/SVM_Calc/MDSA/SVPWM/vIntp_PWMFOC_CalTriCompValue/CalTabc/Cal_TabcValue/CalTabcValue ==
  note: 占空比
  Bus_T1T2_Adjusted_IN : Inport
  Bus_Ts_Vdc : Inport  Port=2
  Add : Sum  Inputs=+--
  Add1 : Sum
  Add2 : Sum
  Bus Creator : BusCreator  Inputs=3
  Bus Selector : BusSelector  OutputSignals=signal1,signal2
  Bus Selector1 : BusSelector  OutputSignals=signal1
  Bus Selector2 : BusSelector  OutputSignals=signal2
  Bus Selector3 : BusSelector  OutputSignals=Ts
  Bus Selector4 : BusSelector  OutputSignals=Ts
  Bus_Ts_Vdc2 : InportShadow  Port=2
  Data Type Conversion1 : DataTypeConversion
  Divide : Product  Inputs=*/
  Divide1 : Product  Inputs=*/
  Divide2 : Product  Inputs=*/
  Gain : Gain  Gain=1/4
  Gain1 : Gain  Gain=0.5
  Gain2 : Gain  Gain=0.5
  Gain3 : Gain  Gain=2
  Gain4 : Gain  Gain=2
  Gain5 : Gain  Gain=2
  Subtract : Sum  Inputs=+-
  Subtract1 : Sum  Inputs=+-
  Subtract2 : Sum  Inputs=+-
  Bus_Tabc : Outport  Description=高电平计数值
  wires:
  Bus Creator/1 -> Bus_Tabc/1
  [Tbon] -> Add2/1
  Bus Selector2/1 -> Gain2/1  "<signal2>"
  [Taon] -> Add1/1
  Bus Selector1/1 -> Gain1/1  "<signal1>"
  Add/1 -> Gain/1
  Bus Selector/2 -> Add/3  "<signal2>"
  Bus Selector/1 -> Add/2  "<signal1>"
  Bus Selector3/1 -> Data Type Conversion1/1  "<Ts>"
  Bus_T1T2_Adjusted_IN/1 -> Bus Selector/1, Bus Selector1/1, Bus Selector2/1
  Data Type Conversion1/1 -> Add/1
  Gain/1 -> Gain3/1, [Taon]
  Gain1/1 -> Add1/2
  Gain2/1 -> Add2/2
  Add1/1 -> Gain4/1, [Tbon]
  Add2/1 -> Gain5/1
  Gain3/1 -> Subtract/2
  Gain4/1 -> Subtract1/2
  Gain5/1 -> Subtract2/2
  Bus Selector4/1 -> Subtract1/1, Divide2/2, Subtract2/1, Divide1/2, Divide/2, Subtract/1  "<Ts>"
  Subtract1/1 -> Divide1/1
  Subtract/1 -> Divide/1
  Subtract2/1 -> Divide2/1
  Divide1/1 -> Bus Creator/2
  Divide/1 -> Bus Creator/1
  Divide2/1 -> Bus Creator/3
  Bus_Ts_Vdc/1 -> Bus Selector3/1
  Bus_Ts_Vdc2/1 -> Bus Selector4/1

== system MDCC/DoCurCtr_sys/MDCC/SVM_Calc/MDSA/SVPWM/vIntp_PWMFOC_CalTriCompValue/CalTabc/Cal_TabcValue/ManageT1T2 ==
  Bus_T1T2_IN : Inport
  Bus_Ts_Vdc : Inport  Port=2
  Add : Sum
  Bus Creator : BusCreator  Inputs=2
  Bus Selector : BusSelector  OutputSignals=signal1,signal2
  Bus Selector1 : BusSelector  OutputSignals=signal1,signal2
  Bus Selector2 : BusSelector  OutputSignals=signal1,signal2
  Bus Selector3 : BusSelector  OutputSignals=Ts
  Constant1 : Constant
  Data Type Conversion : DataTypeConversion
  Data Type Conversion1 : DataTypeConversion
  Divide : Product  Inputs=*/
  Relational Operator : RelationalOperator  Operator=>  OutDataTypeStr=boolean  RndMeth=Nearest
  Signal Conversion : SignalConversion  OverrideOpt=off
  Signal Conversion1 : SignalConversion  OverrideOpt=off
  Subsystem : Subsystem
  Switch : Switch  Criteria=u2 ~= 0  OutDataTypeStr=single  ZeroCross=off
  Switch1 : Switch  Criteria=u2 ~= 0  OutDataTypeStr=single  ZeroCross=off
  Bus_T1T2_Adjusted : Outport
  wires:
  Relational Operator/1 -> Switch1/2, Switch/2
  Divide/1 -> Relational Operator/2
  Add/1 -> Relational Operator/1
  Data Type Conversion1/1 -> Divide/1
  Data Type Conversion/1 -> Divide/2
  Constant1/1 -> Data Type Conversion/1
  Bus Selector/2 -> Add/2  "<signal2>"
  Bus Selector/1 -> Add/1  "<signal1>"
  Bus_T1T2_IN/1 -> Signal Conversion/1, Bus Selector/1, Signal Conversion1/1
  Signal Conversion1/1 -> Subsystem/1(Bus_T1T2_IN)
  Signal Conversion/1 -> Bus Selector1/1
  Subsystem/1(Out1) -> Bus Selector2/1
  Bus Selector1/1 -> Switch/3  "<signal1>"
  Bus Selector2/1 -> Switch/1  "<signal1>"
  Switch/1 -> Bus Creator/1
  Bus Selector2/2 -> Switch1/1  "<signal2>"
  Bus Selector1/2 -> Switch1/3  "<signal2>"
  Switch1/1 -> Bus Creator/2
  Bus Creator/1 -> Bus_T1T2_Adjusted/1
  Bus_Ts_Vdc/1 -> [Bus_Ts_Vdc_ManageT1T2]
  [Bus_Ts_Vdc_ManageT1T2] -> Bus Selector3/1
  Bus Selector3/1 -> Data Type Conversion1/1  "<Ts>"
  [Bus_Ts_Vdc_ManageT1T2] -> Subsystem/2(Bus_Ts_Vdc)

== system MDCC/DoCurCtr_sys/MDCC/UdUqCalc_Sys/MDCC_MCF_Sys/Enabled Subsystem/Harmonic_Injection_11/Subsystem/Harm_11Step_KpKi/Harm11_KpKi_Table ==
  Rdc_absnWoFlt_rads : Inport
  1-D Lookup Table : Lookup_n-D  NumberOfTableDimensions=1  BreakpointsForDimension1=KfMDCC_MCF_Harmonic1113_KpKi_Spd_rads  Table=KfMDCC_MCF_Harmonic11_Kp_coef  InternalRulePriority=Speed  RndMeth=Simplest  InputSameDT=on
  1-D Lookup Table1 : Lookup_n-D  NumberOfTableDimensions=1  BreakpointsForDimension1=KfMDCC_MCF_Harmonic1113_KpKi_Spd_rads  Table=KfMDCC_MCF_Harmonic11_Ki_coef  InternalRulePriority=Speed  RndMeth=Simplest  InputSameDT=on
  Gain : Gain  Gain=0.11e-4
  MCF_Harm11_Kp : Outport  VectorParamsAs1DForOutWhenUnconnected=off
  MCF_Harm11_Ki : Outport  Port=2  VectorParamsAs1DForOutWhenUnconnected=off
  wires:
  1-D Lookup Table/1 -> MCF_Harm11_Kp/1
  1-D Lookup Table1/1 -> Gain/1
  Rdc_absnWoFlt_rads/1 -> 1-D Lookup Table1/1, 1-D Lookup Table/1
  Gain/1 -> MCF_Harm11_Ki/1

== system MDCC/DoCurCtr_sys/MDCC/UdUqCalc_Sys/MDCC_MCF_Sys/Enabled Subsystem/Harmonic_Injection_11/Subsystem/Harm_11Step_KpKi/Harm_11Step_daxis_PI ==
  MCF_Harm_isdDes11 : Inport
  MCF_Harm_isdAct11 : Inport  Port=2
  MCF_Harm_Kp : Inport  Port=3
  MCF_Harm_Ki : Inport  Port=4
  MCF_flgHarm11PIRest : Inport  Port=5
  Add : Sum  Inputs=+-
  Add1 : Sum  Inputs=+-
  Add2 : Sum  Inputs=+++
  Constant : Constant  Value=0  OutDataTypeStr=single
  Constant1 : Constant  Value=-KfMDCC_MCF_HarmonicInUDesMax_V
  Constant3 : Constant  Value=KfMDCC_MCF_HarmonicInUDesMax_V
  Product : Product
  Product1 : Product
  Saturation : simulink/Discontinuities/Saturation Dynamic  OutMin=[]  OutMax=[]  OutDataTypeStr=Inherit: Same as second input  OutDataType=fixdt(1, 16)  OutScaling=2^-10  DoSatur=off
      link override Data Type Propagation: ValuesUsedBestPrec=[11 -11]
  Switch : Switch  Criteria=u2 ~= 0
  Unit Delay : UnitDelay  SampleTime=-1  HasFrameUpgradeWarning=on
  Unit Delay1 : UnitDelay  SampleTime=-1  HasFrameUpgradeWarning=on
  MCF_Harm_ud11PI : Outport  VectorParamsAs1DForOutWhenUnconnected=off
  wires:
  MCF_Harm_isdAct11/1 -> Add/2
  MCF_Harm_isdDes11/1 -> Add/1
  MCF_Harm_Ki/1 -> Product1/2
  Switch/1 -> Add2/3
  Product/1 -> Add2/1
  Product1/1 -> Add2/2
  MCF_Harm_Kp/1 -> Product/2
  Add1/1 -> Product/1
  Unit Delay/1 -> Add1/2
  Add/1 -> Add1/1, Unit Delay/1, Product1/1
  Add2/1 -> Saturation/2
  Saturation/1 -> Unit Delay1/1, MCF_Harm_ud11PI/1
  Constant3/1 -> Saturation/1
  Constant1/1 -> Saturation/3
  MCF_flgHarm11PIRest/1 -> Switch/2
  Constant/1 -> Switch/3
  Unit Delay1/1 -> Switch/1

== system MDCC/DoCurCtr_sys/MDCC/UdUqCalc_Sys/MDCC_MCF_Sys/Enabled Subsystem/Harmonic_Injection_11/Subsystem/Harm_11Step_KpKi/Harm_11Step_qaxis_PI ==
  MCF_Harm_isqDes11 : Inport
  MCF_Harm_isqAct11 : Inport  Port=2
  MCF_Harm_Kp : Inport  Port=3
  MCF_Harm_Ki : Inport  Port=4
  MCF_flgHarm11PIRest : Inport  Port=5
  Add : Sum  Inputs=+-
  Add1 : Sum  Inputs=+-
  Add2 : Sum  Inputs=+++
  Constant : Constant  Value=0  OutDataTypeStr=single
  Constant1 : Constant  Value=-KfMDCC_MCF_HarmonicInUDesMax_V
  Constant3 : Constant  Value=KfMDCC_MCF_HarmonicInUDesMax_V
  Product : Product
  Product1 : Product
  Saturation : simulink/Discontinuities/Saturation Dynamic  OutMin=[]  OutMax=[]  OutDataTypeStr=Inherit: Same as second input  OutDataType=fixdt(1, 16)  OutScaling=2^-10  DoSatur=off
      link override Data Type Propagation: ValuesUsedBestPrec=[11 -11]
  Switch : Switch  Criteria=u2 ~= 0
  Unit Delay : UnitDelay  SampleTime=-1  HasFrameUpgradeWarning=on
  Unit Delay2 : UnitDelay  SampleTime=-1  HasFrameUpgradeWarning=on
  MCF_Harm_uq11PI : Outport  VectorParamsAs1DForOutWhenUnconnected=off
  wires:
  Add/1 -> Product1/1, Unit Delay/1, Add1/1
  Unit Delay/1 -> Add1/2
  Add1/1 -> Product/1
  MCF_Harm_Kp/1 -> Product/2
  Product1/1 -> Add2/2
  Product/1 -> Add2/1
  MCF_Harm_Ki/1 -> Product1/2
  MCF_Harm_isqDes11/1 -> Add/1
  MCF_Harm_isqAct11/1 -> Add/2
  Constant1/1 -> Saturation/3
  Add2/1 -> Saturation/2
  Constant3/1 -> Saturation/1
  MCF_flgHarm11PIRest/1 -> Switch/2
  Saturation/1 -> Unit Delay2/1, MCF_Harm_uq11PI/1
  Switch/1 -> Add2/3
  Constant/1 -> Switch/3
  Unit Delay2/1 -> Switch/1

== system MDCC/DoCurCtr_sys/MDCC/UdUqCalc_Sys/MDCC_MCF_Sys/Enabled Subsystem/Harmonic_Injection_13/Subsystem/Harm_13Step_KpKi/Harm13_KpKi_Table ==
  Rdc_absnWoFlt_rads : Inport
  1-D Lookup Table : Lookup_n-D  NumberOfTableDimensions=1  BreakpointsForDimension1=KfMDCC_MCF_Harmonic1113_KpKi_Spd_rads  Table=KfMDCC_MCF_Harmonic13_Kp_coef  InternalRulePriority=Speed  RndMeth=Simplest  InputSameDT=on
  1-D Lookup Table1 : Lookup_n-D  NumberOfTableDimensions=1  BreakpointsForDimension1=KfMDCC_MCF_Harmonic1113_KpKi_Spd_rads  Table=KfMDCC_MCF_Harmonic13_Ki_coef  InternalRulePriority=Speed  RndMeth=Simplest  InputSameDT=on
  Gain : Gain  Gain=0.13e-4
  MCF_Harm13_Kp : Outport  VectorParamsAs1DForOutWhenUnconnected=off
  MCF_Harm13_Ki : Outport  Port=2  VectorParamsAs1DForOutWhenUnconnected=off
  wires:
  1-D Lookup Table/1 -> MCF_Harm13_Kp/1
  1-D Lookup Table1/1 -> Gain/1
  Rdc_absnWoFlt_rads/1 -> 1-D Lookup Table1/1, 1-D Lookup Table/1
  Gain/1 -> MCF_Harm13_Ki/1

== system MDCC/DoCurCtr_sys/MDCC/UdUqCalc_Sys/MDCC_MCF_Sys/Enabled Subsystem/Harmonic_Injection_13/Subsystem/Harm_13Step_KpKi/Harm_13Step_daxis_PI ==
  MCF_Harm_isdDes13 : Inport
  MCF_Harm_isdAct13 : Inport  Port=2
  MCF_Harm_Kp : Inport  Port=3
  MCF_Harm_Ki : Inport  Port=4
  MCF_flgHarm13PIRest : Inport  Port=5
  Add : Sum  Inputs=+-
  Add1 : Sum  Inputs=+-
  Add2 : Sum  Inputs=+++
  Constant : Constant  Value=0  OutDataTypeStr=single
  Constant1 : Constant  Value=-KfMDCC_MCF_HarmonicInUDesMax_V
  Constant3 : Constant  Value=KfMDCC_MCF_HarmonicInUDesMax_V
  Product : Product
  Product1 : Product
  Saturation : simulink/Discontinuities/Saturation Dynamic  OutMin=[]  OutMax=[]  OutDataTypeStr=Inherit: Same as second input  OutDataType=fixdt(1, 16)  OutScaling=2^-10  DoSatur=off
      link override Data Type Propagation: ValuesUsedBestPrec=[13 -13]
  Switch : Switch  Criteria=u2 ~= 0
  Unit Delay : UnitDelay  SampleTime=-1  HasFrameUpgradeWarning=on
  Unit Delay1 : UnitDelay  SampleTime=-1  HasFrameUpgradeWarning=on
  MCF_Harm_ud13PI : Outport  VectorParamsAs1DForOutWhenUnconnected=off
  wires:
  MCF_Harm_isdAct13/1 -> Add/2
  MCF_Harm_isdDes13/1 -> Add/1
  MCF_Harm_Ki/1 -> Product1/2
  Switch/1 -> Add2/3
  Product/1 -> Add2/1
  Product1/1 -> Add2/2
  MCF_Harm_Kp/1 -> Product/2
  Add1/1 -> Product/1
  Unit Delay/1 -> Add1/2
  Add/1 -> Add1/1, Unit Delay/1, Product1/1
  Add2/1 -> Saturation/2
  Saturation/1 -> Unit Delay1/1, MCF_Harm_ud13PI/1
  Constant3/1 -> Saturation/1
  Constant1/1 -> Saturation/3
  MCF_flgHarm13PIRest/1 -> Switch/2
  Constant/1 -> Switch/3
  Unit Delay1/1 -> Switch/1

== system MDCC/DoCurCtr_sys/MDCC/UdUqCalc_Sys/MDCC_MCF_Sys/Enabled Subsystem/Harmonic_Injection_13/Subsystem/Harm_13Step_KpKi/Harm_13Step_qaxis_PI ==
  MCF_Harm_isqDes13 : Inport
  MCF_Harm_isqAct13 : Inport  Port=2
  MCF_Harm_Kp : Inport  Port=3
  MCF_Harm_Ki : Inport  Port=4
  MCF_flgHarm13PIRest : Inport  Port=5
  Add : Sum  Inputs=+-
  Add1 : Sum  Inputs=+-
  Add2 : Sum  Inputs=+++
  Constant : Constant  Value=0  OutDataTypeStr=single
  Constant1 : Constant  Value=-KfMDCC_MCF_HarmonicInUDesMax_V
  Constant3 : Constant  Value=KfMDCC_MCF_HarmonicInUDesMax_V
  Product : Product
  Product1 : Product
  Saturation : simulink/Discontinuities/Saturation Dynamic  OutMin=[]  OutMax=[]  OutDataTypeStr=Inherit: Same as second input  OutDataType=fixdt(1, 16)  OutScaling=2^-10  DoSatur=off
      link override Data Type Propagation: ValuesUsedBestPrec=[13 -13]
  Switch : Switch  Criteria=u2 ~= 0
  Unit Delay : UnitDelay  SampleTime=-1  HasFrameUpgradeWarning=on
  Unit Delay2 : UnitDelay  SampleTime=-1  HasFrameUpgradeWarning=on
  MCF_Harm_uq13PI : Outport  VectorParamsAs1DForOutWhenUnconnected=off
  wires:
  Add/1 -> Product1/1, Unit Delay/1, Add1/1
  Unit Delay/1 -> Add1/2
  Add1/1 -> Product/1
  MCF_Harm_Kp/1 -> Product/2
  Product1/1 -> Add2/2
  Product/1 -> Add2/1
  MCF_Harm_Ki/1 -> Product1/2
  MCF_Harm_isqDes13/1 -> Add/1
  MCF_Harm_isqAct13/1 -> Add/2
  Constant1/1 -> Saturation/3
  Add2/1 -> Saturation/2
  Constant3/1 -> Saturation/1
  MCF_flgHarm13PIRest/1 -> Switch/2
  Saturation/1 -> Unit Delay2/1, MCF_Harm_uq13PI/1
  Switch/1 -> Add2/3
  Constant/1 -> Switch/3
  Unit Delay2/1 -> Switch/1

== system MDCC/DoCurCtr_sys/MDCC/UdUqCalc_Sys/MDCC_MCF_Sys/Enabled Subsystem/Harmonic_Injection_5/Subsystem/Harm_5Step_KpKi/Harm5_KpKi_Table ==
  Rdc_absnWoFlt_rads : Inport
  1-D Lookup Table : Lookup_n-D  NumberOfTableDimensions=1  BreakpointsForDimension1=KfMDCC_MCF_Harmonic57_KpKi_Spd_rads  Table=KfMDCC_MCF_Harmonic5_Kp_coef  InternalRulePriority=Speed  RndMeth=Simplest  InputSameDT=on
  1-D Lookup Table1 : Lookup_n-D  NumberOfTableDimensions=1  BreakpointsForDimension1=KfMDCC_MCF_Harmonic57_KpKi_Spd_rads  Table=KfMDCC_MCF_Harmonic5_Ki_coef  InternalRulePriority=Speed  RndMeth=Simplest  InputSameDT=on
  Gain : Gain  Gain=0.5e-4
  MCF_Harm5_Kp : Outport  VectorParamsAs1DForOutWhenUnconnected=off
  MCF_Harm5_Ki : Outport  Port=2  VectorParamsAs1DForOutWhenUnconnected=off
  wires:
  1-D Lookup Table/1 -> MCF_Harm5_Kp/1
  1-D Lookup Table1/1 -> Gain/1
  Rdc_absnWoFlt_rads/1 -> 1-D Lookup Table1/1, 1-D Lookup Table/1
  Gain/1 -> MCF_Harm5_Ki/1

== system MDCC/DoCurCtr_sys/MDCC/UdUqCalc_Sys/MDCC_MCF_Sys/Enabled Subsystem/Harmonic_Injection_5/Subsystem/Harm_5Step_KpKi/Harm_5Step_daxis_PI ==
  MCF_Harm_isdDes5 : Inport
  MCF_Harm_isdAct5 : Inport  Port=2
  MCF_Harm_Kp : Inport  Port=3
  MCF_Harm_Ki : Inport  Port=4
  MCF_flgHarm5PIRest : Inport  Port=5
  Add : Sum  Inputs=+-
  Add1 : Sum  Inputs=+-
  Add2 : Sum  Inputs=+++
  Constant : Constant  Value=0  OutDataTypeStr=single
  Constant1 : Constant  Value=-KfMDCC_MCF_HarmonicInUDesMax_V
  Constant3 : Constant  Value=KfMDCC_MCF_HarmonicInUDesMax_V
  Product : Product
  Product1 : Product
  Saturation : simulink/Discontinuities/Saturation Dynamic  OutMin=[]  OutMax=[]  OutDataTypeStr=Inherit: Same as second input  OutDataType=fixdt(1, 16)  OutScaling=2^-10  DoSatur=off
  Switch : Switch  Criteria=u2 ~= 0
  Unit Delay : UnitDelay  SampleTime=-1  HasFrameUpgradeWarning=on
  Unit Delay1 : UnitDelay  SampleTime=-1  HasFrameUpgradeWarning=on
  MCF_Harm_ud5PI : Outport  VectorParamsAs1DForOutWhenUnconnected=off
  wires:
  MCF_Harm_isdAct5/1 -> Add/2
  MCF_Harm_isdDes5/1 -> Add/1
  MCF_Harm_Ki/1 -> Product1/2
  Switch/1 -> Add2/3
  Product/1 -> Add2/1
  Product1/1 -> Add2/2
  MCF_Harm_Kp/1 -> Product/2
  Add1/1 -> Product/1
  Unit Delay/1 -> Add1/2
  Add/1 -> Add1/1, Unit Delay/1, Product1/1
  Add2/1 -> Saturation/2
  Saturation/1 -> Unit Delay1/1, MCF_Harm_ud5PI/1
  Constant3/1 -> Saturation/1
  Constant1/1 -> Saturation/3
  MCF_flgHarm5PIRest/1 -> Switch/2
  Constant/1 -> Switch/3
  Unit Delay1/1 -> Switch/1

== system MDCC/DoCurCtr_sys/MDCC/UdUqCalc_Sys/MDCC_MCF_Sys/Enabled Subsystem/Harmonic_Injection_5/Subsystem/Harm_5Step_KpKi/Harm_5Step_qaxis_PI ==
  MCF_Harm_isqDes5 : Inport
  MCF_Harm_isqAct5 : Inport  Port=2
  MCF_Harm_Kp : Inport  Port=3
  MCF_Harm_Ki : Inport  Port=4
  MCF_flgHarm5PIRest : Inport  Port=5
  Add : Sum  Inputs=+-
  Add1 : Sum  Inputs=+-
  Add2 : Sum  Inputs=+++
  Constant : Constant  Value=0  OutDataTypeStr=single
  Constant1 : Constant  Value=-KfMDCC_MCF_HarmonicInUDesMax_V
  Constant3 : Constant  Value=KfMDCC_MCF_HarmonicInUDesMax_V
  Product : Product
  Product1 : Product
  Saturation : simulink/Discontinuities/Saturation Dynamic  OutMin=[]  OutMax=[]  OutDataTypeStr=Inherit: Same as second input  OutDataType=fixdt(1, 16)  OutScaling=2^-10  DoSatur=off
  Switch : Switch  Criteria=u2 ~= 0
  Unit Delay : UnitDelay  SampleTime=-1  HasFrameUpgradeWarning=on
  Unit Delay2 : UnitDelay  SampleTime=-1  HasFrameUpgradeWarning=on
  MCF_Harm_uq5PI : Outport  VectorParamsAs1DForOutWhenUnconnected=off
  wires:
  Add/1 -> Product1/1, Unit Delay/1, Add1/1
  Unit Delay/1 -> Add1/2
  Add1/1 -> Product/1
  MCF_Harm_Kp/1 -> Product/2
  Product1/1 -> Add2/2
  Product/1 -> Add2/1
  MCF_Harm_Ki/1 -> Product1/2
  MCF_Harm_isqDes5/1 -> Add/1
  MCF_Harm_isqAct5/1 -> Add/2
  Constant1/1 -> Saturation/3
  Add2/1 -> Saturation/2
  Constant3/1 -> Saturation/1
  MCF_flgHarm5PIRest/1 -> Switch/2
  Saturation/1 -> Unit Delay2/1, MCF_Harm_uq5PI/1
  Switch/1 -> Add2/3
  Constant/1 -> Switch/3
  Unit Delay2/1 -> Switch/1

== system MDCC/DoCurCtr_sys/MDCC/UdUqCalc_Sys/MDCC_MCF_Sys/Enabled Subsystem/Harmonic_Injection_7/Subsystem/Harm_7Step_KpKi/Harm7_KpKi_Table ==
  Rdc_absnWoFlt_rads : Inport
  1-D Lookup Table : Lookup_n-D  NumberOfTableDimensions=1  BreakpointsForDimension1=KfMDCC_MCF_Harmonic57_KpKi_Spd_rads  Table=KfMDCC_MCF_Harmonic7_Kp_coef  InternalRulePriority=Speed  RndMeth=Simplest  InputSameDT=on
  1-D Lookup Table1 : Lookup_n-D  NumberOfTableDimensions=1  BreakpointsForDimension1=KfMDCC_MCF_Harmonic57_KpKi_Spd_rads  Table=KfMDCC_MCF_Harmonic7_Ki_coef  InternalRulePriority=Speed  RndMeth=Simplest  InputSameDT=on
  Gain : Gain  Gain=0.7e-4
  MCF_Harm7_Kp : Outport  VectorParamsAs1DForOutWhenUnconnected=off
  MCF_Harm7_Ki : Outport  Port=2  VectorParamsAs1DForOutWhenUnconnected=off
  wires:
  1-D Lookup Table/1 -> MCF_Harm7_Kp/1
  1-D Lookup Table1/1 -> Gain/1
  Rdc_absnWoFlt_rads/1 -> 1-D Lookup Table1/1, 1-D Lookup Table/1
  Gain/1 -> MCF_Harm7_Ki/1

== system MDCC/DoCurCtr_sys/MDCC/UdUqCalc_Sys/MDCC_MCF_Sys/Enabled Subsystem/Harmonic_Injection_7/Subsystem/Harm_7Step_KpKi/Harm_7Step_daxis_PI ==
  MCF_Harm_isdDes7 : Inport
  MCF_Harm_isdAct7 : Inport  Port=2
  MCF_Harm_Kp : Inport  Port=3
  MCF_Harm_Ki : Inport  Port=4
  MCF_flgHarm7PIRest : Inport  Port=5
  Add : Sum  Inputs=+-
  Add1 : Sum  Inputs=+-
  Add2 : Sum  Inputs=+++
  Constant : Constant  Value=0  OutDataTypeStr=single
  Constant1 : Constant  Value=-KfMDCC_MCF_HarmonicInUDesMax_V
  Constant3 : Constant  Value=KfMDCC_MCF_HarmonicInUDesMax_V
  Product : Product
  Product1 : Product
  Saturation : simulink/Discontinuities/Saturation Dynamic  OutMin=[]  OutMax=[]  OutDataTypeStr=Inherit: Same as second input  OutDataType=fixdt(1, 16)  OutScaling=2^-10  DoSatur=off
      link override Data Type Propagation: ValuesUsedBestPrec=[7 -7]
  Switch : Switch  Criteria=u2 ~= 0
  Unit Delay : UnitDelay  SampleTime=-1  HasFrameUpgradeWarning=on
  Unit Delay1 : UnitDelay  SampleTime=-1  HasFrameUpgradeWarning=on
  MCF_Harm_ud7PI : Outport  VectorParamsAs1DForOutWhenUnconnected=off
  wires:
  MCF_Harm_isdAct7/1 -> Add/2
  MCF_Harm_isdDes7/1 -> Add/1
  MCF_Harm_Ki/1 -> Product1/2
  Switch/1 -> Add2/3
  Product/1 -> Add2/1
  Product1/1 -> Add2/2
  MCF_Harm_Kp/1 -> Product/2
  Add1/1 -> Product/1
  Unit Delay/1 -> Add1/2
  Add/1 -> Add1/1, Unit Delay/1, Product1/1
  Add2/1 -> Saturation/2
  Saturation/1 -> Unit Delay1/1, MCF_Harm_ud7PI/1
  Constant3/1 -> Saturation/1
  Constant1/1 -> Saturation/3
  MCF_flgHarm7PIRest/1 -> Switch/2
  Constant/1 -> Switch/3
  Unit Delay1/1 -> Switch/1

== system MDCC/DoCurCtr_sys/MDCC/UdUqCalc_Sys/MDCC_MCF_Sys/Enabled Subsystem/Harmonic_Injection_7/Subsystem/Harm_7Step_KpKi/Harm_7Step_qaxis_PI ==
  MCF_Harm_isqDes7 : Inport
  MCF_Harm_isqAct7 : Inport  Port=2
  MCF_Harm_Kp : Inport  Port=3
  MCF_Harm_Ki : Inport  Port=4
  MCF_flgHarm7PIRest : Inport  Port=5
  Add : Sum  Inputs=+-
  Add1 : Sum  Inputs=+-
  Add2 : Sum  Inputs=+++
  Constant : Constant  Value=0  OutDataTypeStr=single
  Constant1 : Constant  Value=-KfMDCC_MCF_HarmonicInUDesMax_V
  Constant3 : Constant  Value=KfMDCC_MCF_HarmonicInUDesMax_V
  Product : Product
  Product1 : Product
  Saturation : simulink/Discontinuities/Saturation Dynamic  OutMin=[]  OutMax=[]  OutDataTypeStr=Inherit: Same as second input  OutDataType=fixdt(1, 16)  OutScaling=2^-10  DoSatur=off
      link override Data Type Propagation: ValuesUsedBestPrec=[7 -7]
  Switch : Switch  Criteria=u2 ~= 0
  Unit Delay : UnitDelay  SampleTime=-1  HasFrameUpgradeWarning=on
  Unit Delay2 : UnitDelay  SampleTime=-1  HasFrameUpgradeWarning=on
  MCF_Harm_uq7PI : Outport  VectorParamsAs1DForOutWhenUnconnected=off
  wires:
  Add/1 -> Product1/1, Unit Delay/1, Add1/1
  Unit Delay/1 -> Add1/2
  Add1/1 -> Product/1
  MCF_Harm_Kp/1 -> Product/2
  Product1/1 -> Add2/2
  Product/1 -> Add2/1
  MCF_Harm_Ki/1 -> Product1/2
  MCF_Harm_isqDes7/1 -> Add/1
  MCF_Harm_isqAct7/1 -> Add/2
  Constant1/1 -> Saturation/3
  Add2/1 -> Saturation/2
  Constant3/1 -> Saturation/1
  MCF_flgHarm7PIRest/1 -> Switch/2
  Saturation/1 -> Unit Delay2/1, MCF_Harm_uq7PI/1
  Switch/1 -> Add2/3
  Constant/1 -> Switch/3
  Unit Delay2/1 -> Switch/1

== system MDCC/DoCurCtr_sys/MDCC/SVM_Calc/MDSA/SVPWM/vIntp_PWMFOC_CalTriCompValue/CalTabc/Cal_TabcValue/ManageT1T2/Subsystem ==
  Bus_T1T2_IN : Inport
  Bus_Ts_Vdc : Inport  Port=2
  Add : Sum
  Bus Creator : BusCreator  Inputs=2
  Bus Selector : BusSelector  OutputSignals=signal1,signal2
  Bus Selector1 : BusSelector  OutputSignals=Ts
  Divide : Product  Inputs=*/
  Divide1 : Product  Inputs=*/
  Gain : Gain  Commented=on  Gain=Ts
  Gain1 : Gain  Commented=on  Gain=Ts
  Product : Product
  Product1 : Product
  Out1 : Outport
  wires:
  Bus Creator/1 -> Out1/1
  [Bus_T1T2_T2] -> Divide1/1
  Add/1 -> Divide1/2, Divide/2
  Bus Selector/2 -> Add/2, [Bus_T1T2_T2]  "<signal2>"
  Bus Selector/1 -> Add/1, Divide/1  "<signal1>"
  Bus_T1T2_IN/1 -> Bus Selector/1
  Bus_Ts_Vdc/1 -> Bus Selector1/1
  Bus Selector1/1 -> Product1/2, Product/2  "<Ts>"
  Divide1/1 -> Product/1
  Product/1 -> Bus Creator/2
  Divide/1 -> Product1/1
  Product1/1 -> Bus Creator/1
